simulink model "TCMSSystem"  (R2019b)
settings: configuration reference "ConfigSet_TCMSSystem_Reference" (kept outside this file)
model workspace (MAT data in the model file):
  Prm_TCMSSystem : Simulink.Parameter (value not decoded)
  SampleTime = 0.05
symbols that are objects in the model workspace (value not decoded): Prm_TCMSSystem
undefined symbols (not defined in the file): ADDIntervention, AK1Status, AK2Status, AKContactorStatus, AllDoorsClosed, AllLeftDoorsClosed, AllRightDoorsClosed, APS1Fault, APS1Isolated, APS1OutputVoltage, APS1Status, APS2Fault, APS2Isolated, APS2OutputVoltage, APS2Status, APSKAKContactor, ASCOEnd1, ASCOEnd2, ATBMode, ATCBypassMode, ATCStatusNotOK, ATOMode, ATPLowSpeedCutoutStatus, ATPMode, AuxCompressor, BatteryCurrent, BatteryIsolationContactor, BatteryTemperature, BatteryVoltage, BCG1Fault, BCG1Isolated, BCG1IsolationFailed, BCG1OutputCurrent, BCG1Status, BCG2Fault, BCG2Isolated, BCG2OutputCurrent, BCG2Status, BCGOutputVoltage, BECU1AxleLockedWheelSet1, BECU2AxleLockedWheelSet2, BECUFaulty, BECUMajorFault, BECUMinorFault, BECUStatus, BIC1Inside, BIC1Outside, BIC2Inside, BIC2Outside, Bogie, Bogie1WSPStatus, Bogie2WSPStatus, BogieFaulty, BogieIsolationStatus, BogieSupportedMass, BrakeCylinderPressureGauge, BrakeLoopCBTripped, BrakeLoopOpenTL, BrakeTrainLineStatus, BrakingDemand ... (+215)
libraries: TimersLib x257, simulink x137, LatchesLib x42, VectorOperationsLib x15, TestBenchLib x12, MathOperationsLib x2, FiltersLib x1
(part 9 of 16)

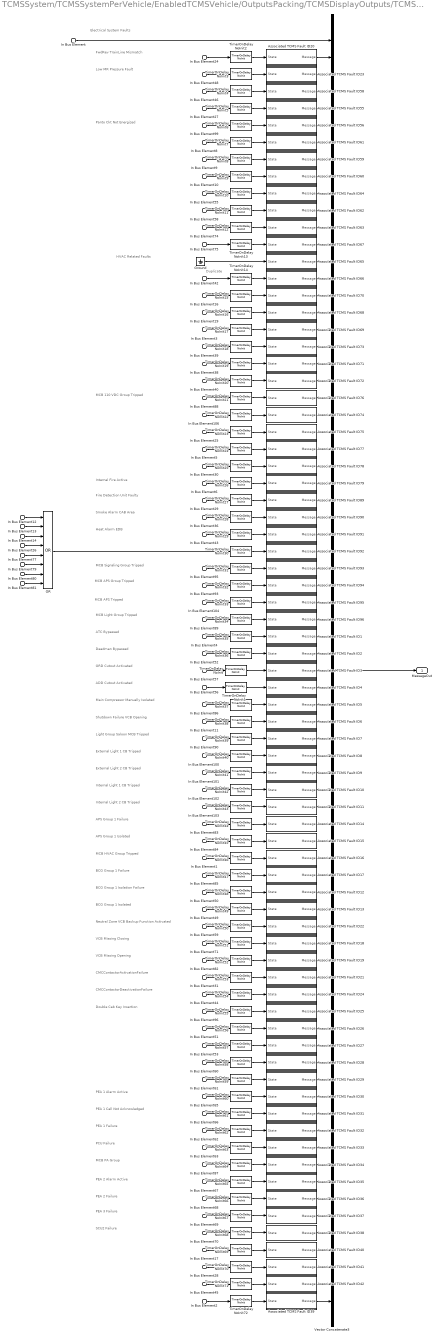
== system TCMSSystem/TCMSSystemPerVehicle/EnabledTCMSVehicle/OutputsPacking/TCMSDisplayOutputs/TCMSMessageEvents/ElectricalSystemFaults ==
  note: Duplicate
  note: FwdRev TrainLine Mismatch
  note: Low MR Pressure Fault
  note: Electrical System Faults
  note: ATC Bypassed
  note: Deadman Bypassed
  note: ORD Cutout Activated
  note: ADD Cutout Activated
  note: Main Compressor Manually Isolated
  note: Shutdown Failure VCB Opening
  note: Light Group Saloon MCB Tripped
  note: External Light 1 CB Tripped
  note: External Light 2 CB Tripped
  note: Internal Light 1 CB Tripped
  note: Internal Light 2 CB Tripped
  note: APS Group 1 Failure
  note: APS Group 1 Isolated
  note: MCB HVAC Group Tripped
  note: BCG Group 1 Failure
  note: BCG Group 1 Isolation Failure
  note: BCG Group 1 Isolated
  note: Neutral Zone VCB Backup Function Activated
  note: VCB Missing Closing
  note: VCB Missing Opening
  note: CMCContactorActivationFailure
  note: CMCContactorDeactivationFailure
  note: Double Cab Key Insertion
  note: PEA 1 Alarm Active
  note: PEA 1 Call Not Acknowledged
  note: PEA 1 Failure
  note: PCU Failure
  note: MCB PA Group
  note: PEA 2 Alarm Active
  note: PEA 2 Failure
  note: PEA 3 Failure
  note: SCU2 Failure
  note: MCB Light Group Tripped
  note: MCB APS Group Tripped
  note: MCB Signaling Group Tripped
  note: MCB 110 VDC Group Tripped
  note: Panto Ckt Not Energized
  note: MCB APS Tripped
  note: Internal Fire Active
  note: Fire Detection Unit Faulty
  note: Smoke Alarm CAB Area
  note: Heat Alarm EDB
  note: HVAC Related Faults
  In Bus Element : Inport  PortName=MessageIn
  In Bus Element4 : Inport  Port=2  PortName=BusIn  Element=ElectricalSystem.ATCBypassMode
  In Bus Element3 : Inport  Port=2  PortName=BusIn  Element=ElectricalSystem.RCCBTripped
  In Bus Element38 : Inport  Port=2  PortName=BusIn  Element=ElectricalSystem.ExtSmokeDetectedinHVAC
  In Bus Element39 : Inport  Port=2  PortName=BusIn  Element=ElectricalSystem.HVACFireMode
  In Bus Element40 : Inport  Port=2  PortName=BusIn  Element=ElectricalSystem.HVACReducedMode
  In Bus Element42 : Inport  Port=2  PortName=BusIn  Element=ElectricalSystem.HVACMajorFault
  In Bus Element16 : Inport  Port=2  PortName=BusIn  Element=ElectricalSystem.SupplyFanTripped
  In Bus Element19 : Inport  Port=2  PortName=BusIn  Element=ElectricalSystem.EmergencyInverterTripped
  In Bus Element36 : Inport  Port=2  PortName=BusIn  Element=ElectricalSystem.SmokeAlarmCABArea
  In Bus Element43 : Inport  Port=2  PortName=BusIn  Element=ElectricalSystem.HeatAlarmEDB
  In Bus Element29 : Inport  Port=2  PortName=BusIn  Element=ElectricalSystem.FDUFault
  In Bus Element6 : Inport  Port=2  PortName=BusIn  Element=ElectricalSystem.InternalFire
  In Bus Element49 : Inport  Port=2  PortName=BusIn  Element=ElectricalSystem.BCG1Isolated
  In Bus Element50 : Inport  Port=2  PortName=BusIn  Element=ElectricalSystem.BCG1IsolationFailed
  In Bus Element83 : Inport  Port=2  PortName=BusIn  Element=ElectricalSystem.APS1Fault
  In Bus Element84 : Inport  Port=2  PortName=BusIn  Element=ElectricalSystem.APS1Isolated
  In Bus Element85 : Inport  Port=2  PortName=BusIn  Element=ElectricalSystem.BCG1Fault
  In Bus Element1 : Inport  Port=2  PortName=BusIn  Element=ElectricalSystem.HVACGroupMCBTripped
  In Bus Element12 : Inport  Port=2  PortName=BusIn  Element=DoorSystem.Doors.DoorA1UnexpectedOpen
  In Bus Element13 : Inport  Port=2  PortName=BusIn  Element=DoorSystem.Doors.DoorA2UnexpectedOpen
  In Bus Element14 : Inport  Port=2  PortName=BusIn  Element=DoorSystem.Doors.DoorA3UnexpectedOpen
  In Bus Element26 : Inport  Port=2  PortName=BusIn  Element=DoorSystem.Doors.DoorA4UnexpectedOpen
  In Bus Element77 : Inport  Port=2  PortName=BusIn  Element=DoorSystem.Doors.DoorB1UnexpectedOpen
  In Bus Element79 : Inport  Port=2  PortName=BusIn  Element=DoorSystem.Doors.DoorB2UnexpectedOpen
  In Bus Element80 : Inport  Port=2  PortName=BusIn  Element=DoorSystem.Doors.DoorB3UnexpectedOpen
  In Bus Element81 : Inport  Port=2  PortName=BusIn  Element=DoorSystem.Doors.DoorB4UnexpectedOpen
  In Bus Element8 : Inport  Port=3  PortName=VehicleLevelFaults  Element=PantographPipeLowPressure
  In Bus Element9 : Inport  Port=3  PortName=VehicleLevelFaults  Element=TransformerOilPressureTooLow
  In Bus Element10 : Inport  Port=3  PortName=VehicleLevelFaults  Element=TransformerOilTemperatureTooHigh
  In Bus Element25 : Inport  Port=3  PortName=VehicleLevelFaults  Element=BatteryFuseBlown
  In Bus Element51 : Inport  Port=3  PortName=VehicleLevelFaults  Element=TransformerOilLevelLow
  In Bus Element53 : Inport  Port=3  PortName=VehicleLevelFaults  Element=TransformerOilFlowWarning
  In Bus Element60 : Inport  Port=3  PortName=VehicleLevelFaults  Element=TransformerOilPressureWarning
  In Bus Element61 : Inport  Port=3  PortName=VehicleLevelFaults  Element=TransformerOilTemperatureHigh
  In Bus Element62 : Inport  Port=3  PortName=VehicleLevelFaults  Element=PEA1Failure
  In Bus Element63 : Inport  Port=3  PortName=VehicleLevelFaults  Element=PCUFailure
  In Bus Element65 : Inport  Port=3  PortName=VehicleLevelFaults  Element=PEA1AlarmActive
  In Bus Element66 : Inport  Port=3  PortName=VehicleLevelFaults  Element=PEA1CallNotAcknowledged
  In Bus Element67 : Inport  Port=3  PortName=VehicleLevelFaults  Element=PEA2AlarmActive
  In Bus Element68 : Inport  Port=3  PortName=VehicleLevelFaults  Element=PEA2Failure
  In Bus Element69 : Inport  Port=3  PortName=VehicleLevelFaults  Element=PEA3Failure
  In Bus Element70 : Inport  Port=3  PortName=VehicleLevelFaults  Element=SCU2Failure
  In Bus Element2 : Inport  Port=3  PortName=VehicleLevelFaults  Element=TransformerOilLevelTooLow
  In Bus Element59 : Inport  Port=4  PortName=ElectricalControl  Element=NeutralZoneBackupModeActive
  In Bus Element30 : Inport  Port=4  PortName=ElectricalControl  Element=BatteryLowFault
  In Bus Element27 : Inport  Port=4  PortName=ElectricalControl  Element=BUVDR_Active
  In Bus Element31 : Inport  Port=4  PortName=ElectricalControl  Element=CMCActivationFault
  In Bus Element44 : Inport  Port=4  PortName=ElectricalControl  Element=CMCDeactivationFault
  In Bus Element46 : Inport  Port=4  PortName=ElectricalControl  Element=VCBOpenedByCI
  In Bus Element55 : Inport  Port=4  PortName=ElectricalControl  Element=VCBOpenedByACOvercurrent
  In Bus Element58 : Inport  Port=4  PortName=ElectricalControl  Element=VCBOpenedByMTrProtection
  In Bus Element74 : Inport  Port=4  PortName=ElectricalControl  Element=VCBOpenedByAPS
  In Bus Element5 : Inport  Port=4  PortName=ElectricalControl  Element=BICContactorActivationFault
  In Bus Element11 : Inport  Port=4  PortName=ElectricalControl  Element=ShutdownFailureVCBNotOpening
  In Bus Element17 : Inport  Port=4  PortName=ElectricalControl  Element=PantographRisingMissing
  In Bus Element28 : Inport  Port=4  PortName=ElectricalControl  Element=PantographLoweringMissing
  In Bus Element45 : Inport  Port=4  PortName=ElectricalControl  Element=PantographRisingInhibited
  In Bus Element75 : Inport  Port=4  PortName=ElectricalControl  Element=PantographLoweringFailure
  In Bus Element71 : Inport  Port=4  PortName=ElectricalControl  Element=VCBMissingClosing
  In Bus Element82 : Inport  Port=4  PortName=ElectricalControl  Element=VCBMissingOpening
  In Bus Element24 : Inport  Port=4  PortName=ElectricalControl  Element=FwdRevTrainLineMismatchMessage
  In Bus Element48 : Inport  Port=4  PortName=ElectricalControl  Element=LowMRPressureFaultMessage
  In Bus Element52 : Inport  Port=4  PortName=ElectricalControl  Element=DeadmanBypass
  In Bus Element56 : Inport  Port=4  PortName=ElectricalControl  Element=ADDCOSStatus
  In Bus Element57 : Inport  Port=4  PortName=ElectricalControl  Element=ORDCOSStatus
  In Bus Element86 : Inport  Port=4  PortName=ElectricalControl  Element=AirSupplyIC
  In Bus Element87 : Inport  Port=4  PortName=ElectricalControl  Element=MCBPAGroupStatus
  In Bus Element88 : Inport  Port=4  PortName=ElectricalControl  Element=MCB110VDCGroup
  In Bus Element89 : Inport  Port=4  PortName=ElectricalControl  Element=MCBLightGroup
  In Bus Element90 : Inport  Port=4  PortName=ElectricalControl  Element=MCBLightSaloonGroup
  In Bus Element93 : Inport  Port=4  PortName=ElectricalControl  Element=MCBAPSGroup
  In Bus Element95 : Inport  Port=4  PortName=ElectricalControl  Element=MCBSignallingGroup
  In Bus Element96 : Inport  Port=4  PortName=ElectricalControl  Element=DoubleCabKeyInsertion
  In Bus Element99 : Inport  Port=4  PortName=ElectricalControl  Element=PantoCircuitNotEnergized
  In Bus Element100 : Inport  Port=4  PortName=ElectricalControl  Element=ExternalLightCB1Tripped
  In Bus Element101 : Inport  Port=4  PortName=ElectricalControl  Element=ExternalLightCB2Tripped
  In Bus Element102 : Inport  Port=4  PortName=ElectricalControl  Element=InternalLightCB1Tripped
  In Bus Element103 : Inport  Port=4  PortName=ElectricalControl  Element=InternalLightCB2Tripped
  In Bus Element104 : Inport  Port=4  PortName=ElectricalControl  Element=APSCBTripped
  In Bus Element106 : Inport  Port=4  PortName=ElectricalControl  Element=MCDRFaulty
  Associated TCMS Fault ID1 : Subsystem  mask{MessageID=120001}
      mask Display:
      | port_label('output', 1, ['ID = ' num2str(MessageID)])
      | port_label('input', 1, 'Status')
  Associated TCMS Fault ID10 : Subsystem  mask{MessageID=112005}
      mask Display:
      | port_label('output', 1, ['ID = ' num2str(MessageID)])
      | port_label('input', 1, 'Status')
  Associated TCMS Fault ID11 : Subsystem  mask{MessageID=113006}
      mask Display:
      | port_label('output', 1, ['ID = ' num2str(MessageID)])
      | port_label('input', 1, 'Status')
  Associated TCMS Fault ID12 : Subsystem  mask{MessageID=223003}
      mask Display:
      | port_label('output', 1, ['ID = ' num2str(MessageID)])
      | port_label('input', 1, 'Status')
  Associated TCMS Fault ID13 : Subsystem  mask{MessageID=223005}
      mask Display:
      | port_label('output', 1, ['ID = ' num2str(MessageID)])
      | port_label('input', 1, 'Status')
  Associated TCMS Fault ID14 : Subsystem  mask{MessageID=232002}
      mask Display:
      | port_label('output', 1, ['ID = ' num2str(MessageID)])
      | port_label('input', 1, 'Status')
  Associated TCMS Fault ID15 : Subsystem  mask{MessageID=232004}
      mask Display:
      | port_label('output', 1, ['ID = ' num2str(MessageID)])
      | port_label('input', 1, 'Status')
  Associated TCMS Fault ID16 : Subsystem  mask{MessageID=081001}
      mask Display:
      | port_label('output', 1, ['ID = ' num2str(MessageID)])
      | port_label('input', 1, 'Status')
  Associated TCMS Fault ID17 : Subsystem  mask{MessageID=223001}
      mask Display:
      | port_label('output', 1, ['ID = ' num2str(MessageID)])
      | port_label('input', 1, 'Status')
  Associated TCMS Fault ID18 : Subsystem  mask{MessageID=012024}
      mask Display:
      | port_label('output', 1, ['ID = ' num2str(MessageID)])
      | port_label('input', 1, 'Status')
  Associated TCMS Fault ID19 : Subsystem  mask{MessageID=012025}
      mask Display:
      | port_label('output', 1, ['ID = ' num2str(MessageID)])
      | port_label('input', 1, 'Status')
  Associated TCMS Fault ID2 : Subsystem  mask{MessageID=001008}
      mask Display:
      | port_label('output', 1, ['ID = ' num2str(MessageID)])
      | port_label('input', 1, 'Status')
  Associated TCMS Fault ID20 : Subsystem  mask{MessageID=031032}
      mask Display:
      | port_label('output', 1, ['ID = ' num2str(MessageID)])
      | port_label('input', 1, 'Status')
  Associated TCMS Fault ID21 : Subsystem  mask{MessageID=021004}
      mask Display:
      | port_label('output', 1, ['ID = ' num2str(MessageID)])
      | port_label('input', 1, 'Status')
  Associated TCMS Fault ID22 : Subsystem  mask{MessageID=241006}
      mask Display:
      | port_label('output', 1, ['ID = ' num2str(MessageID)])
      | port_label('input', 1, 'Status')
  Associated TCMS Fault ID23 : Subsystem  mask{MessageID=091007}
      mask Display:
      | port_label('output', 1, ['ID = ' num2str(MessageID)])
      | port_label('input', 1, 'Status')
  Associated TCMS Fault ID24 : Subsystem  mask{MessageID=021003}
      mask Display:
      | port_label('output', 1, ['ID = ' num2str(MessageID)])
      | port_label('input', 1, 'Status')
  Associated TCMS Fault ID25 : Subsystem  mask{MessageID=030018}
      mask Display:
      | port_label('output', 1, ['ID = ' num2str(MessageID)])
      | port_label('input', 1, 'Status')
  Associated TCMS Fault ID26 : Subsystem  mask{MessageID=012008}
      mask Display:
      | port_label('output', 1, ['ID = ' num2str(MessageID)])
      | port_label('input', 1, 'Status')
  Associated TCMS Fault ID27 : Subsystem  mask{MessageID=012011}
      mask Display:
      | port_label('output', 1, ['ID = ' num2str(MessageID)])
      | port_label('input', 1, 'Status')
  Associated TCMS Fault ID28 : Subsystem  mask{MessageID=012012}
      mask Display:
      | port_label('output', 1, ['ID = ' num2str(MessageID)])
      | port_label('input', 1, 'Status')
  Associated TCMS Fault ID29 : Subsystem  mask{MessageID=012026}
      mask Display:
      | port_label('output', 1, ['ID = ' num2str(MessageID)])
      | port_label('input', 1, 'Status')
  Associated TCMS Fault ID3 : Subsystem  mask{MessageID=012103}
      mask Display:
      | port_label('output', 1, ['ID = ' num2str(MessageID)])
      | port_label('input', 1, 'Status')
  Associated TCMS Fault ID30 : Subsystem  mask{MessageID=131001}
      mask Display:
      | port_label('output', 1, ['ID = ' num2str(MessageID)])
      | port_label('input', 1, 'Status')
  Associated TCMS Fault ID31 : Subsystem  mask{MessageID=131005}
      mask Display:
      | port_label('output', 1, ['ID = ' num2str(MessageID)])
      | port_label('input', 1, 'Status')
  Associated TCMS Fault ID32 : Subsystem  mask{MessageID=131010}
      mask Display:
      | port_label('output', 1, ['ID = ' num2str(MessageID)])
      | port_label('input', 1, 'Status')
  Associated TCMS Fault ID33 : Subsystem  mask{MessageID=131014}
      mask Display:
      | port_label('output', 1, ['ID = ' num2str(MessageID)])
      | port_label('input', 1, 'Status')
  Associated TCMS Fault ID34 : Subsystem  mask{MessageID=131015}
      mask Display:
      | port_label('output', 1, ['ID = ' num2str(MessageID)])
      | port_label('input', 1, 'Status')
  Associated TCMS Fault ID35 : Subsystem  mask{MessageID=133002}
      mask Display:
      | port_label('output', 1, ['ID = ' num2str(MessageID)])
      | port_label('input', 1, 'Status')
  Associated TCMS Fault ID36 : Subsystem  mask{MessageID=131011}
      mask Display:
      | port_label('output', 1, ['ID = ' num2str(MessageID)])
      | port_label('input', 1, 'Status')
  Associated TCMS Fault ID37 : Subsystem  mask{MessageID=131012}
      mask Display:
      | port_label('output', 1, ['ID = ' num2str(MessageID)])
      | port_label('input', 1, 'Status')
  Associated TCMS Fault ID38 : Subsystem  mask{MessageID=132009}
      mask Display:
      | port_label('output', 1, ['ID = ' num2str(MessageID)])
      | port_label('input', 1, 'Status')
  Associated TCMS Fault ID39 : Subsystem  mask{MessageID=012009}
      mask Display:
      | port_label('output', 1, ['ID = ' num2str(MessageID)])
      | port_label('input', 1, 'Status')
  Associated TCMS Fault ID4 : Subsystem  mask{MessageID=012104}
      mask Display:
      | port_label('output', 1, ['ID = ' num2str(MessageID)])
      | port_label('input', 1, 'Status')
  Associated TCMS Fault ID40 : Subsystem  mask{MessageID=012019}
      mask Display:
      | port_label('output', 1, ['ID = ' num2str(MessageID)])
      | port_label('input', 1, 'Status')
  Associated TCMS Fault ID41 : Subsystem  mask{MessageID=012020}
      mask Display:
      | port_label('output', 1, ['ID = ' num2str(MessageID)])
      | port_label('input', 1, 'Status')
  Associated TCMS Fault ID42 : Subsystem  mask{MessageID=012023}
      mask Display:
      | port_label('output', 1, ['ID = ' num2str(MessageID)])
      | port_label('input', 1, 'Status')
  Associated TCMS Fault ID5 : Subsystem  mask{MessageID=021001}
      mask Display:
      | port_label('output', 1, ['ID = ' num2str(MessageID)])
      | port_label('input', 1, 'Status')
  Associated TCMS Fault ID55 : Subsystem  mask{MessageID=012003}
      mask Display:
      | port_label('output', 1, ['ID = ' num2str(MessageID)])
      | port_label('input', 1, 'Status')
  Associated TCMS Fault ID56 : Subsystem  mask{MessageID=012005}
      mask Display:
      | port_label('output', 1, ['ID = ' num2str(MessageID)])
      | port_label('input', 1, 'Status')
  Associated TCMS Fault ID58 : Subsystem  mask{MessageID=011017}
      mask Display:
      | port_label('output', 1, ['ID = ' num2str(MessageID)])
      | port_label('input', 1, 'Status')
  Associated TCMS Fault ID59 : Subsystem  mask{MessageID=012010}
      mask Display:
      | port_label('output', 1, ['ID = ' num2str(MessageID)])
      | port_label('input', 1, 'Status')
  Associated TCMS Fault ID6 : Subsystem  mask{MessageID=000014}
      mask Display:
      | port_label('output', 1, ['ID = ' num2str(MessageID)])
      | port_label('input', 1, 'Status')
  Associated TCMS Fault ID60 : Subsystem  mask{MessageID=012013}
      mask Display:
      | port_label('output', 1, ['ID = ' num2str(MessageID)])
      | port_label('input', 1, 'Status')
  Associated TCMS Fault ID61 : Subsystem  mask{MessageID=012006}
      mask Display:
      | port_label('output', 1, ['ID = ' num2str(MessageID)])
      | port_label('input', 1, 'Status')
  Associated TCMS Fault ID62 : Subsystem  mask{MessageID=012016}
      mask Display:
      | port_label('output', 1, ['ID = ' num2str(MessageID)])
      | port_label('input', 1, 'Status')
  Associated TCMS Fault ID63 : Subsystem  mask{MessageID=012018}
      mask Display:
      | port_label('output', 1, ['ID = ' num2str(MessageID)])
      | port_label('input', 1, 'Status')
  Associated TCMS Fault ID64 : Subsystem  mask{MessageID=012015}
      mask Display:
      | port_label('output', 1, ['ID = ' num2str(MessageID)])
      | port_label('input', 1, 'Status')
  Associated TCMS Fault ID65 : Subsystem  mask{MessageID=081001}
      mask Display:
      | port_label('output', 1, ['ID = ' num2str(MessageID)])
      | port_label('input', 1, 'Status')
  Associated TCMS Fault ID66 : Subsystem  mask{MessageID=081010}
      mask Display:
      | port_label('output', 1, ['ID = ' num2str(MessageID)])
      | port_label('input', 1, 'Status')
  Associated TCMS Fault ID67 : Subsystem  mask{MessageID=012022}
      mask Display:
      | port_label('output', 1, ['ID = ' num2str(MessageID)])
      | port_label('input', 1, 'Status')
  Associated TCMS Fault ID68 : Subsystem  mask{MessageID=081012}
      mask Display:
      | port_label('output', 1, ['ID = ' num2str(MessageID)])
      | port_label('input', 1, 'Status')
  Associated TCMS Fault ID69 : Subsystem  mask{MessageID=081013}
      mask Display:
      | port_label('output', 1, ['ID = ' num2str(MessageID)])
      | port_label('input', 1, 'Status')
  Associated TCMS Fault ID7 : Subsystem  mask{MessageID=111002}
      mask Display:
      | port_label('output', 1, ['ID = ' num2str(MessageID)])
      | port_label('input', 1, 'Status')
  Associated TCMS Fault ID70 : Subsystem  mask{MessageID=081011}
      mask Display:
      | port_label('output', 1, ['ID = ' num2str(MessageID)])
      | port_label('input', 1, 'Status')
  Associated TCMS Fault ID71 : Subsystem  mask{MessageID=081015}
      mask Display:
      | port_label('output', 1, ['ID = ' num2str(MessageID)])
      | port_label('input', 1, 'Status')
  Associated TCMS Fault ID72 : Subsystem  mask{MessageID=081016}
      mask Display:
      | port_label('output', 1, ['ID = ' num2str(MessageID)])
      | port_label('input', 1, 'Status')
  Associated TCMS Fault ID73 : Subsystem  mask{MessageID=081014}
      mask Display:
      | port_label('output', 1, ['ID = ' num2str(MessageID)])
      | port_label('input', 1, 'Status')
  Associated TCMS Fault ID74 : Subsystem  mask{MessageID=031034}
      mask Display:
      | port_label('output', 1, ['ID = ' num2str(MessageID)])
      | port_label('input', 1, 'Status')
  Associated TCMS Fault ID75 : Subsystem  mask{MessageID=033005}
      mask Display:
      | port_label('output', 1, ['ID = ' num2str(MessageID)])
      | port_label('input', 1, 'Status')
  Associated TCMS Fault ID76 : Subsystem  mask{MessageID=031029}
      mask Display:
      | port_label('output', 1, ['ID = ' num2str(MessageID)])
      | port_label('input', 1, 'Status')
  Associated TCMS Fault ID77 : Subsystem  mask{MessageID=033007}
      mask Display:
      | port_label('output', 1, ['ID = ' num2str(MessageID)])
      | port_label('input', 1, 'Status')
  Associated TCMS Fault ID78 : Subsystem  mask{MessageID=033031}
      mask Display:
      | port_label('output', 1, ['ID = ' num2str(MessageID)])
      | port_label('input', 1, 'Status')
  Associated TCMS Fault ID79 : Subsystem  mask{MessageID=150500}
      mask Display:
      | port_label('output', 1, ['ID = ' num2str(MessageID)])
      | port_label('input', 1, 'Status')
  Associated TCMS Fault ID8 : Subsystem  mask{MessageID=112003}
      mask Display:
      | port_label('output', 1, ['ID = ' num2str(MessageID)])
      | port_label('input', 1, 'Status')
  Associated TCMS Fault ID89 : Subsystem  mask{MessageID=150502}
      mask Display:
      | port_label('output', 1, ['ID = ' num2str(MessageID)])
      | port_label('input', 1, 'Status')
  Associated TCMS Fault ID9 : Subsystem  mask{MessageID=113004}
      mask Display:
      | port_label('output', 1, ['ID = ' num2str(MessageID)])
      | port_label('input', 1, 'Status')
  Associated TCMS Fault ID90 : Subsystem  mask{MessageID=151004}
      mask Display:
      | port_label('output', 1, ['ID = ' num2str(MessageID)])
      | port_label('input', 1, 'Status')
  Associated TCMS Fault ID91 : Subsystem  mask{MessageID=151021}
      mask Display:
      | port_label('output', 1, ['ID = ' num2str(MessageID)])
      | port_label('input', 1, 'Status')
  Associated TCMS Fault ID92 : Subsystem  mask{MessageID=120003}
      mask Display:
      | port_label('output', 1, ['ID = ' num2str(MessageID)])
      | port_label('input', 1, 'Status')
  Associated TCMS Fault ID93 : Subsystem  mask{MessageID=121004}
      mask Display:
      | port_label('output', 1, ['ID = ' num2str(MessageID)])
      | port_label('input', 1, 'Status')
  Associated TCMS Fault ID94 : Subsystem  mask{MessageID=232001}
      mask Display:
      | port_label('output', 1, ['ID = ' num2str(MessageID)])
      | port_label('input', 1, 'Status')
  Associated TCMS Fault ID95 : Subsystem  mask{MessageID=232158}
      mask Display:
      | port_label('output', 1, ['ID = ' num2str(MessageID)])
      | port_label('input', 1, 'Status')
  Associated TCMS Fault ID96 : Subsystem  mask{MessageID=111001}
      mask Display:
      | port_label('output', 1, ['ID = ' num2str(MessageID)])
      | port_label('input', 1, 'Status')
  Ground : Ground
  OR : Logic  Operator=OR  Inputs=8  AllPortsSameDT=off  OutDataTypeStr=boolean
  TimerOnDelay NoInit{,1..72} (73 alike) : TimersLib/TimerOnDelay NoInit  UpperSaturationLimit=0.5  OutputTime=off  SampleTime=-1
      settings: SourceProductName=Sydac Utilities
  Vector Concatenate3 : Concatenate  NumInputs=75
  MessageOut : Outport
  wires:
  Associated TCMS Fault ID70/1(Message) -> Vector Concatenate3/16
  Associated TCMS Fault ID63/1(Message) -> Vector Concatenate3/12
  Associated TCMS Fault ID58/1(Message) -> Vector Concatenate3/4
  Associated TCMS Fault ID23/1(Message) -> Vector Concatenate3/3
  Associated TCMS Fault ID64/1(Message) -> Vector Concatenate3/10
  Associated TCMS Fault ID96/1(Message) -> Vector Concatenate3/35
  Associated TCMS Fault ID67/1(Message) -> Vector Concatenate3/13
  Associated TCMS Fault ID90/1(Message) -> Vector Concatenate3/29
  Associated TCMS Fault ID77/1(Message) -> Vector Concatenate3/25
  Associated TCMS Fault ID20/1(Message) -> Vector Concatenate3/2
  Associated TCMS Fault ID89/1(Message) -> Vector Concatenate3/28
  Associated TCMS Fault ID76/1(Message) -> Vector Concatenate3/22
  Associated TCMS Fault ID79/1(Message) -> Vector Concatenate3/27
  Associated TCMS Fault ID71/1(Message) -> Vector Concatenate3/20
  Associated TCMS Fault ID69/1(Message) -> Vector Concatenate3/18
  Associated TCMS Fault ID95/1(Message) -> Vector Concatenate3/34
  Associated TCMS Fault ID74/1(Message) -> Vector Concatenate3/23
  Associated TCMS Fault ID65/1(Message) -> Vector Concatenate3/14
  Associated TCMS Fault ID92/1(Message) -> Vector Concatenate3/31
  Associated TCMS Fault ID73/1(Message) -> Vector Concatenate3/19
  Associated TCMS Fault ID72/1(Message) -> Vector Concatenate3/21
  Associated TCMS Fault ID61/1(Message) -> Vector Concatenate3/7
  Associated TCMS Fault ID55/1(Message) -> Vector Concatenate3/5
  Associated TCMS Fault ID91/1(Message) -> Vector Concatenate3/30
  Associated TCMS Fault ID56/1(Message) -> Vector Concatenate3/6
  Associated TCMS Fault ID93/1(Message) -> Vector Concatenate3/32
  Associated TCMS Fault ID60/1(Message) -> Vector Concatenate3/9
  In Bus Element24/1 -> TimerOnDelay NoInit2/1
  Associated TCMS Fault ID78/1(Message) -> Vector Concatenate3/26
  Associated TCMS Fault ID62/1(Message) -> Vector Concatenate3/11
  Associated TCMS Fault ID68/1(Message) -> Vector Concatenate3/17
  Associated TCMS Fault ID75/1(Message) -> Vector Concatenate3/24
  Associated TCMS Fault ID94/1(Message) -> Vector Concatenate3/33
  Associated TCMS Fault ID59/1(Message) -> Vector Concatenate3/8
  Associated TCMS Fault ID66/1(Message) -> Vector Concatenate3/15
  In Bus Element48/1 -> TimerOnDelay NoInit3/1
  Vector Concatenate3/1 -> MessageOut/1
  In Bus Element/1 -> Vector Concatenate3/1
  In Bus Element46/1 -> TimerOnDelay NoInit4/1
  In Bus Element27/1 -> TimerOnDelay NoInit5/1
  In Bus Element99/1 -> TimerOnDelay NoInit6/1
  In Bus Element8/1 -> TimerOnDelay NoInit7/1
  In Bus Element9/1 -> TimerOnDelay NoInit8/1
  In Bus Element10/1 -> TimerOnDelay NoInit9/1
  In Bus Element55/1 -> TimerOnDelay NoInit10/1
  In Bus Element58/1 -> TimerOnDelay NoInit11/1
  In Bus Element75/1 -> TimerOnDelay NoInit13/1
  In Bus Element74/1 -> TimerOnDelay NoInit12/1
  Ground/1 -> Associated TCMS Fault ID65/1(State)
  In Bus Element42/1 -> TimerOnDelay NoInit14/1
  In Bus Element40/1 -> TimerOnDelay NoInit20/1
  In Bus Element38/1 -> TimerOnDelay NoInit19/1
  In Bus Element39/1 -> TimerOnDelay NoInit18/1
  In Bus Element3/1 -> TimerOnDelay NoInit17/1
  In Bus Element19/1 -> TimerOnDelay NoInit16/1
  In Bus Element16/1 -> TimerOnDelay NoInit15/1
  In Bus Element88/1 -> TimerOnDelay NoInit21/1
  In Bus Element106/1 -> TimerOnDelay NoInit22/1
  In Bus Element25/1 -> TimerOnDelay NoInit23/1
  In Bus Element5/1 -> TimerOnDelay NoInit24/1
  In Bus Element30/1 -> TimerOnDelay NoInit25/1
  In Bus Element6/1 -> TimerOnDelay NoInit26/1
  In Bus Element29/1 -> TimerOnDelay NoInit27/1
  In Bus Element36/1 -> TimerOnDelay NoInit28/1
  In Bus Element43/1 -> TimerOnDelay NoInit29/1
  OR/1 -> TimerOnDelay NoInit30/1
  In Bus Element95/1 -> TimerOnDelay NoInit31/1
  In Bus Element93/1 -> TimerOnDelay NoInit32/1
  In Bus Element89/1 -> TimerOnDelay NoInit34/1
  In Bus Element4/1 -> TimerOnDelay NoInit35/1
  Associated TCMS Fault ID1/1(Message) -> Vector Concatenate3/36
  Associated TCMS Fault ID2/1(Message) -> Vector Concatenate3/37
  In Bus Element52/1 -> TimerOnDelay NoInit36/1
  In Bus Element56/1 -> TimerOnDelay NoInit1/1
  Associated TCMS Fault ID4/1(Message) -> Vector Concatenate3/39
  Associated TCMS Fault ID3/1(Message) -> Vector Concatenate3/38
  In Bus Element57/1 -> TimerOnDelay NoInit/1
  Associated TCMS Fault ID5/1(Message) -> Vector Concatenate3/40
  In Bus Element86/1 -> TimerOnDelay NoInit37/1
  Associated TCMS Fault ID6/1(Message) -> Vector Concatenate3/41
  Associated TCMS Fault ID7/1(Message) -> Vector Concatenate3/42
  In Bus Element90/1 -> TimerOnDelay NoInit39/1
  In Bus Element100/1 -> TimerOnDelay NoInit40/1
  Associated TCMS Fault ID8/1(Message) -> Vector Concatenate3/43
  Associated TCMS Fault ID9/1(Message) -> Vector Concatenate3/44
  In Bus Element101/1 -> TimerOnDelay NoInit41/1
  In Bus Element102/1 -> TimerOnDelay NoInit42/1
  Associated TCMS Fault ID10/1(Message) -> Vector Concatenate3/45
  Associated TCMS Fault ID11/1(Message) -> Vector Concatenate3/46
  In Bus Element103/1 -> TimerOnDelay NoInit43/1
  In Bus Element49/1 -> TimerOnDelay NoInit49/1
  Associated TCMS Fault ID13/1(Message) -> Vector Concatenate3/52
  Associated TCMS Fault ID12/1(Message) -> Vector Concatenate3/51
  In Bus Element50/1 -> TimerOnDelay NoInit48/1
  In Bus Element85/1 -> TimerOnDelay NoInit47/1
  Associated TCMS Fault ID17/1(Message) -> Vector Concatenate3/50
  Associated TCMS Fault ID16/1(Message) -> Vector Concatenate3/49
  In Bus Element1/1 -> TimerOnDelay NoInit46/1
  In Bus Element84/1 -> TimerOnDelay NoInit45/1
  Associated TCMS Fault ID15/1(Message) -> Vector Concatenate3/48
  Associated TCMS Fault ID14/1(Message) -> Vector Concatenate3/47
  In Bus Element83/1 -> TimerOnDelay NoInit44/1
  Associated TCMS Fault ID22/1(Message) -> Vector Concatenate3/53
  In Bus Element59/1 -> TimerOnDelay NoInit50/1
  In Bus Element71/1 -> TimerOnDelay NoInit51/1
  Associated TCMS Fault ID18/1(Message) -> Vector Concatenate3/54
  Associated TCMS Fault ID19/1(Message) -> Vector Concatenate3/55
  In Bus Element82/1 -> TimerOnDelay NoInit52/1
  In Bus Element44/1 -> TimerOnDelay NoInit54/1
  Associated TCMS Fault ID24/1(Message) -> Vector Concatenate3/57
  Associated TCMS Fault ID21/1(Message) -> Vector Concatenate3/56
  In Bus Element31/1 -> TimerOnDelay NoInit53/1
  In Bus Element96/1 -> TimerOnDelay NoInit55/1
  Associated TCMS Fault ID25/1(Message) -> Vector Concatenate3/58
  Associated TCMS Fault ID26/1(Message) -> Vector Concatenate3/59
  Associated TCMS Fault ID27/1(Message) -> Vector Concatenate3/60
  Associated TCMS Fault ID28/1(Message) -> Vector Concatenate3/61
  Associated TCMS Fault ID29/1(Message) -> Vector Concatenate3/62
  In Bus Element61/1 -> TimerOnDelay NoInit59/1
  In Bus Element60/1 -> TimerOnDelay NoInit58/1
  In Bus Element53/1 -> TimerOnDelay NoInit57/1
  In Bus Element51/1 -> TimerOnDelay NoInit56/1
  In Bus Element67/1 -> TimerOnDelay NoInit65/1
  In Bus Element68/1 -> TimerOnDelay NoInit66/1
  In Bus Element70/1 -> TimerOnDelay NoInit68/1
  Associated TCMS Fault ID38/1(Message) -> Vector Concatenate3/71
  Associated TCMS Fault ID37/1(Message) -> Vector Concatenate3/70
  Associated TCMS Fault ID36/1(Message) -> Vector Concatenate3/69
  Associated TCMS Fault ID35/1(Message) -> Vector Concatenate3/68
  Associated TCMS Fault ID34/1(Message) -> Vector Concatenate3/67
  In Bus Element87/1 -> TimerOnDelay NoInit64/1
  In Bus Element62/1 -> TimerOnDelay NoInit62/1
  Associated TCMS Fault ID32/1(Message) -> Vector Concatenate3/65
  Associated TCMS Fault ID33/1(Message) -> Vector Concatenate3/66
  In Bus Element63/1 -> TimerOnDelay NoInit63/1
  In Bus Element66/1 -> TimerOnDelay NoInit61/1
  Associated TCMS Fault ID31/1(Message) -> Vector Concatenate3/64
  Associated TCMS Fault ID30/1(Message) -> Vector Concatenate3/63
  In Bus Element65/1 -> TimerOnDelay NoInit60/1
  In Bus Element69/1 -> TimerOnDelay NoInit67/1
  In Bus Element11/1 -> TimerOnDelay NoInit38/1
  In Bus Element28/1 -> TimerOnDelay NoInit70/1
  In Bus Element17/1 -> TimerOnDelay NoInit69/1
  In Bus Element45/1 -> TimerOnDelay NoInit71/1
  Associated TCMS Fault ID40/1(Message) -> Vector Concatenate3/72
  Associated TCMS Fault ID41/1(Message) -> Vector Concatenate3/73
  Associated TCMS Fault ID42/1(Message) -> Vector Concatenate3/74
  In Bus Element80/1 -> OR/7
  In Bus Element81/1 -> OR/8
  In Bus Element79/1 -> OR/6
  In Bus Element14/1 -> OR/3
  In Bus Element13/1 -> OR/2
  In Bus Element77/1 -> OR/5
  In Bus Element12/1 -> OR/1
  In Bus Element26/1 -> OR/4
  In Bus Element104/1 -> TimerOnDelay NoInit33/1
  Associated TCMS Fault ID39/1(Message) -> Vector Concatenate3/75
  In Bus Element2/1 -> TimerOnDelay NoInit72/1
  TimerOnDelay NoInit/1 -> Associated TCMS Fault ID3/1(State)
  TimerOnDelay NoInit1/1 -> Associated TCMS Fault ID4/1(State)
  TimerOnDelay NoInit2/1 -> Associated TCMS Fault ID20/1(State)
  TimerOnDelay NoInit3/1 -> Associated TCMS Fault ID23/1(State)
  TimerOnDelay NoInit4/1 -> Associated TCMS Fault ID58/1(State)
  TimerOnDelay NoInit5/1 -> Associated TCMS Fault ID55/1(State)
  TimerOnDelay NoInit6/1 -> Associated TCMS Fault ID56/1(State)
  TimerOnDelay NoInit7/1 -> Associated TCMS Fault ID61/1(State)
  TimerOnDelay NoInit8/1 -> Associated TCMS Fault ID59/1(State)
  TimerOnDelay NoInit9/1 -> Associated TCMS Fault ID60/1(State)
  TimerOnDelay NoInit10/1 -> Associated TCMS Fault ID64/1(State)
  TimerOnDelay NoInit11/1 -> Associated TCMS Fault ID62/1(State)
  TimerOnDelay NoInit12/1 -> Associated TCMS Fault ID63/1(State)
  TimerOnDelay NoInit13/1 -> Associated TCMS Fault ID67/1(State)
  TimerOnDelay NoInit14/1 -> Associated TCMS Fault ID66/1(State)
  TimerOnDelay NoInit15/1 -> Associated TCMS Fault ID70/1(State)
  TimerOnDelay NoInit16/1 -> Associated TCMS Fault ID68/1(State)
  TimerOnDelay NoInit17/1 -> Associated TCMS Fault ID69/1(State)
  TimerOnDelay NoInit18/1 -> Associated TCMS Fault ID73/1(State)
  TimerOnDelay NoInit19/1 -> Associated TCMS Fault ID71/1(State)
  TimerOnDelay NoInit20/1 -> Associated TCMS Fault ID72/1(State)
  TimerOnDelay NoInit21/1 -> Associated TCMS Fault ID76/1(State)
  TimerOnDelay NoInit22/1 -> Associated TCMS Fault ID74/1(State)
  TimerOnDelay NoInit23/1 -> Associated TCMS Fault ID75/1(State)
  TimerOnDelay NoInit24/1 -> Associated TCMS Fault ID77/1(State)
  TimerOnDelay NoInit25/1 -> Associated TCMS Fault ID78/1(State)
  TimerOnDelay NoInit26/1 -> Associated TCMS Fault ID79/1(State)
  TimerOnDelay NoInit27/1 -> Associated TCMS Fault ID89/1(State)
  TimerOnDelay NoInit28/1 -> Associated TCMS Fault ID90/1(State)
  TimerOnDelay NoInit29/1 -> Associated TCMS Fault ID91/1(State)
  TimerOnDelay NoInit30/1 -> Associated TCMS Fault ID92/1(State)
  TimerOnDelay NoInit31/1 -> Associated TCMS Fault ID93/1(State)
  TimerOnDelay NoInit32/1 -> Associated TCMS Fault ID94/1(State)
  TimerOnDelay NoInit33/1 -> Associated TCMS Fault ID95/1(State)
  TimerOnDelay NoInit34/1 -> Associated TCMS Fault ID96/1(State)
  TimerOnDelay NoInit35/1 -> Associated TCMS Fault ID1/1(State)
  TimerOnDelay NoInit36/1 -> Associated TCMS Fault ID2/1(State)
  TimerOnDelay NoInit37/1 -> Associated TCMS Fault ID5/1(State)
  TimerOnDelay NoInit38/1 -> Associated TCMS Fault ID6/1(State)
  TimerOnDelay NoInit39/1 -> Associated TCMS Fault ID7/1(State)
  TimerOnDelay NoInit40/1 -> Associated TCMS Fault ID8/1(State)
  TimerOnDelay NoInit41/1 -> Associated TCMS Fault ID9/1(State)
  TimerOnDelay NoInit42/1 -> Associated TCMS Fault ID10/1(State)
  TimerOnDelay NoInit43/1 -> Associated TCMS Fault ID11/1(State)
  TimerOnDelay NoInit44/1 -> Associated TCMS Fault ID14/1(State)
  TimerOnDelay NoInit45/1 -> Associated TCMS Fault ID15/1(State)
  TimerOnDelay NoInit46/1 -> Associated TCMS Fault ID16/1(State)
  TimerOnDelay NoInit47/1 -> Associated TCMS Fault ID17/1(State)
  TimerOnDelay NoInit48/1 -> Associated TCMS Fault ID12/1(State)
  TimerOnDelay NoInit49/1 -> Associated TCMS Fault ID13/1(State)
  TimerOnDelay NoInit50/1 -> Associated TCMS Fault ID22/1(State)
  TimerOnDelay NoInit51/1 -> Associated TCMS Fault ID18/1(State)
  TimerOnDelay NoInit52/1 -> Associated TCMS Fault ID19/1(State)
  TimerOnDelay NoInit53/1 -> Associated TCMS Fault ID21/1(State)
  TimerOnDelay NoInit54/1 -> Associated TCMS Fault ID24/1(State)
  TimerOnDelay NoInit55/1 -> Associated TCMS Fault ID25/1(State)
  TimerOnDelay NoInit56/1 -> Associated TCMS Fault ID26/1(State)
  TimerOnDelay NoInit57/1 -> Associated TCMS Fault ID27/1(State)
  TimerOnDelay NoInit58/1 -> Associated TCMS Fault ID28/1(State)
  TimerOnDelay NoInit59/1 -> Associated TCMS Fault ID29/1(State)
  TimerOnDelay NoInit60/1 -> Associated TCMS Fault ID30/1(State)
  TimerOnDelay NoInit61/1 -> Associated TCMS Fault ID31/1(State)
  TimerOnDelay NoInit62/1 -> Associated TCMS Fault ID32/1(State)
  TimerOnDelay NoInit63/1 -> Associated TCMS Fault ID33/1(State)
  TimerOnDelay NoInit64/1 -> Associated TCMS Fault ID34/1(State)
  TimerOnDelay NoInit65/1 -> Associated TCMS Fault ID35/1(State)
  TimerOnDelay NoInit66/1 -> Associated TCMS Fault ID36/1(State)
  TimerOnDelay NoInit67/1 -> Associated TCMS Fault ID37/1(State)
  TimerOnDelay NoInit68/1 -> Associated TCMS Fault ID38/1(State)
  TimerOnDelay NoInit69/1 -> Associated TCMS Fault ID40/1(State)
  TimerOnDelay NoInit70/1 -> Associated TCMS Fault ID41/1(State)
  TimerOnDelay NoInit71/1 -> Associated TCMS Fault ID42/1(State)
  TimerOnDelay NoInit72/1 -> Associated TCMS Fault ID39/1(State)

== system TCMSSystem/TCMSSystemPerVehicle/EnabledTCMSVehicle/OutputsPacking/TCMSDisplayOutputs/TCMSMessageEvents/MessageShortList ==
  AllFaults : Inport
  Associated TCMS Fault ID : Subsystem  Commented=on  mask{MessageID=0}
      mask Display:
      | port_label('output', 1, ['ID = ' num2str(MessageID)])
      | port_label('input', 1, 'Status')
  Constant : Constant  Value=0
  For Each Subsystem : Subsystem  TreatAsAtomicUnit=on
  Selector : Selector  IndexMode=Zero-based  IndexOptions=Index vector (port)  Indices=[1 3]  OutputSizes=1
  TCMS Message Index List : Subsystem
  Vector Concatenate : Concatenate
  ActiveFaults : Outport
  wires:
  Selector/1 -> ActiveFaults/1
  TCMS Message Index List/1(IndexList) -> Selector/2
  For Each Subsystem/1(MessageStatus) -> TCMS Message Index List/1(Status)
  AllFaults/1 -> Vector Concatenate/2, For Each Subsystem/1(Message)
  Constant/1 -> Associated TCMS Fault ID/1(State)
  Associated TCMS Fault ID/1(Message) -> Vector Concatenate/1
  Vector Concatenate/1 -> Selector/1

== system TCMSSystem/TCMSSystemPerVehicle/EnabledTCMSVehicle/OutputsPacking/TCMSDisplayOutputs/TCMSMessageEvents/MiscellaneousFaults ==
  note: Miscellaneous
  note: Coupling Circuit Not Energized
  note: Cab Enabling CB Tripped
  In Bus Element : Inport  PortName=MessageIn
  In Bus Element6 : Inport  Port=2  PortName=VehicleLevelFaults  Element=WFLFailure
  In Bus Element7 : Inport  Port=2  PortName=VehicleLevelFaults  Element=TrainRadioFailure
  In Bus Element8 : Inport  Port=3  PortName=BusIn  Element=TCMSSystem.RemoteHornIsolated
  In Bus Element3 : Inport  Port=4  PortName=TractionControl  Element=VehicleDerailed
  In Bus Element5 : Inport  Port=5  PortName=ElectricalControl  Element=CabEnableNotEnergized
  In Bus Element11 : Inport  Port=5  PortName=ElectricalControl  Element=CouplingCircuitNotEnergized
  In Bus Element4 : Inport  Port=5  PortName=ElectricalControl  Element=ObstacleDetected
  In Bus Element9 : Inport  Port=5  PortName=ElectricalControl  Element=ODDFailure
  Associated TCMS Fault ID1 : Subsystem  mask{MessageID=001010}
      mask Display:
      | port_label('output', 1, ['ID = ' num2str(MessageID)])
      | port_label('input', 1, 'Status')
  Associated TCMS Fault ID102 : Subsystem  mask{MessageID=031028}
      mask Display:
      | port_label('output', 1, ['ID = ' num2str(MessageID)])
      | port_label('input', 1, 'Status')
  Associated TCMS Fault ID103 : Subsystem  mask{MessageID=031036}
      mask Display:
      | port_label('output', 1, ['ID = ' num2str(MessageID)])
      | port_label('input', 1, 'Status')
  Associated TCMS Fault ID104 : Subsystem  mask{MessageID=0261001}
      mask Display:
      | port_label('output', 1, ['ID = ' num2str(MessageID)])
      | port_label('input', 1, 'Status')
  Associated TCMS Fault ID105 : Subsystem  mask{MessageID=001002}
      mask Display:
      | port_label('output', 1, ['ID = ' num2str(MessageID)])
      | port_label('input', 1, 'Status')
  Associated TCMS Fault ID106 : Subsystem  mask{MessageID=001003}
      mask Display:
      | port_label('output', 1, ['ID = ' num2str(MessageID)])
      | port_label('input', 1, 'Status')
  Associated TCMS Fault ID107 : Subsystem  mask{MessageID=001001}
      mask Display:
      | port_label('output', 1, ['ID = ' num2str(MessageID)])
      | port_label('input', 1, 'Status')
  Associated TCMS Fault ID108 : Subsystem  mask{MessageID=171001}
      mask Display:
      | port_label('output', 1, ['ID = ' num2str(MessageID)])
      | port_label('input', 1, 'Status')
  TimerOnDelay NoInit{1..8} (8 alike) : TimersLib/TimerOnDelay NoInit  UpperSaturationLimit=0.5  OutputTime=off  SampleTime=-1
      settings: SourceProductName=Sydac Utilities
  Vector Concatenate7 : Concatenate  NumInputs=9
  MessageOut : Outport
  wires:
  Associated TCMS Fault ID104/1(Message) -> Vector Concatenate7/2
  In Bus Element7/1 -> TimerOnDelay NoInit7/1
  Associated TCMS Fault ID108/1(Message) -> Vector Concatenate7/8
  Vector Concatenate7/1 -> MessageOut/1
  Associated TCMS Fault ID106/1(Message) -> Vector Concatenate7/5
  Associated TCMS Fault ID103/1(Message) -> Vector Concatenate7/7
  Associated TCMS Fault ID105/1(Message) -> Vector Concatenate7/4
  Associated TCMS Fault ID107/1(Message) -> Vector Concatenate7/3
  Associated TCMS Fault ID102/1(Message) -> Vector Concatenate7/6
  In Bus Element/1 -> Vector Concatenate7/1
  In Bus Element9/1 -> TimerOnDelay NoInit1/1
  In Bus Element4/1 -> TimerOnDelay NoInit3/1
  In Bus Element3/1 -> TimerOnDelay NoInit4/1
  In Bus Element11/1 -> TimerOnDelay NoInit5/1
  In Bus Element5/1 -> TimerOnDelay NoInit6/1
  In Bus Element6/1 -> TimerOnDelay NoInit2/1
  Associated TCMS Fault ID1/1(Message) -> Vector Concatenate7/9
  In Bus Element8/1 -> TimerOnDelay NoInit8/1
  TimerOnDelay NoInit2/1 -> Associated TCMS Fault ID104/1(State)
  TimerOnDelay NoInit1/1 -> Associated TCMS Fault ID107/1(State)
  TimerOnDelay NoInit3/1 -> Associated TCMS Fault ID105/1(State)
  TimerOnDelay NoInit4/1 -> Associated TCMS Fault ID106/1(State)
  TimerOnDelay NoInit5/1 -> Associated TCMS Fault ID102/1(State)
  TimerOnDelay NoInit6/1 -> Associated TCMS Fault ID103/1(State)
  TimerOnDelay NoInit7/1 -> Associated TCMS Fault ID108/1(State)
  TimerOnDelay NoInit8/1 -> Associated TCMS Fault ID1/1(State)
